simulink model "OCRtest"  (R2023b)
settings: Solver=VariableStepAuto  StartTime=0.0  StopTime=t_stop  RelTol=1e-3
values from neighbouring files (symbols this model uses):
  input_P = P(i)    [Batch_running.m]
  input_T = T(i)    [Batch_running.m]
  input_V = V(i)    [Batch_running.m]
settings Model: Creator=Administrator  LastModifiedBy=Administrator

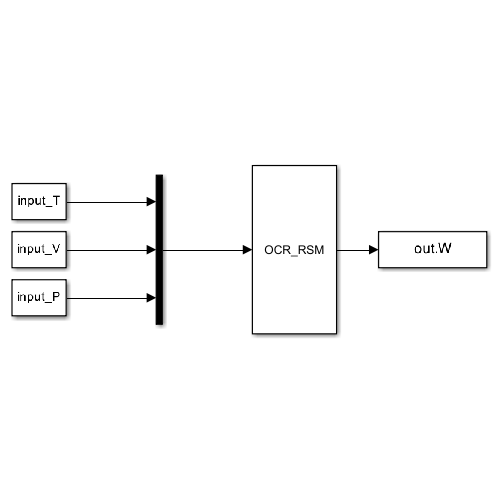
[thumbnail: Simulink's stored preview of the top-level diagram]
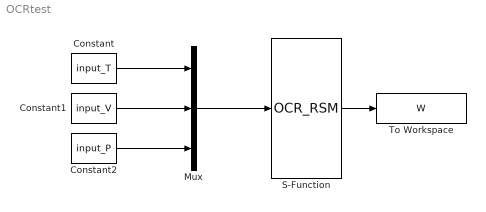
== system OCRtest ==
  Constant : Constant  Value=input_T
  Constant1 : Constant  Value=input_V
  Constant2 : Constant  Value=input_P
  Mux : Mux  Inputs=3
  S-Function : S-Function  FunctionName=OCR_RSM  SFunctionDeploymentMode=off  EnableBusSupport=off
  To Workspace : ToWorkspace  VariableName=W  SampleTime=-1
  wires:
  Mux/1 -> S-Function/1
  Constant/1 -> Mux/1
  Constant1/1 -> Mux/2
  Constant2/1 -> Mux/3
  S-Function/1 -> To Workspace/1
